simulink model "Radial_KID_MPC"  (R2022a)
settings: Solver=FixedStepAuto  StartTime=0.0  StopTime=Tf  FixedStep=Ts  RelTol=1e-3
values from neighbouring files (symbols this model uses):
  eta = 0.001    [vdp_MPC.m]
  Ts = ts    [dataset_join.m]    (also in vdp_Koopman.m = 0.01)
undefined symbols (not defined in the file or in its folder): DiscIntNeverNeededParam
libraries: sharedTrackingLibrary x1, mpclib x1
settings Model: Creator=sergiovaneg  LastModifiedBy=sergiovaneg

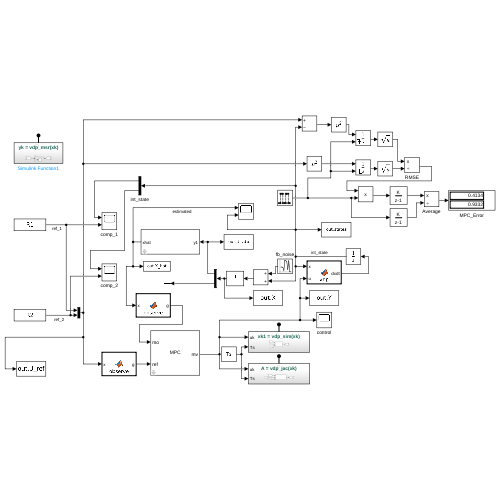
[thumbnail: Simulink's stored preview of the top-level diagram]
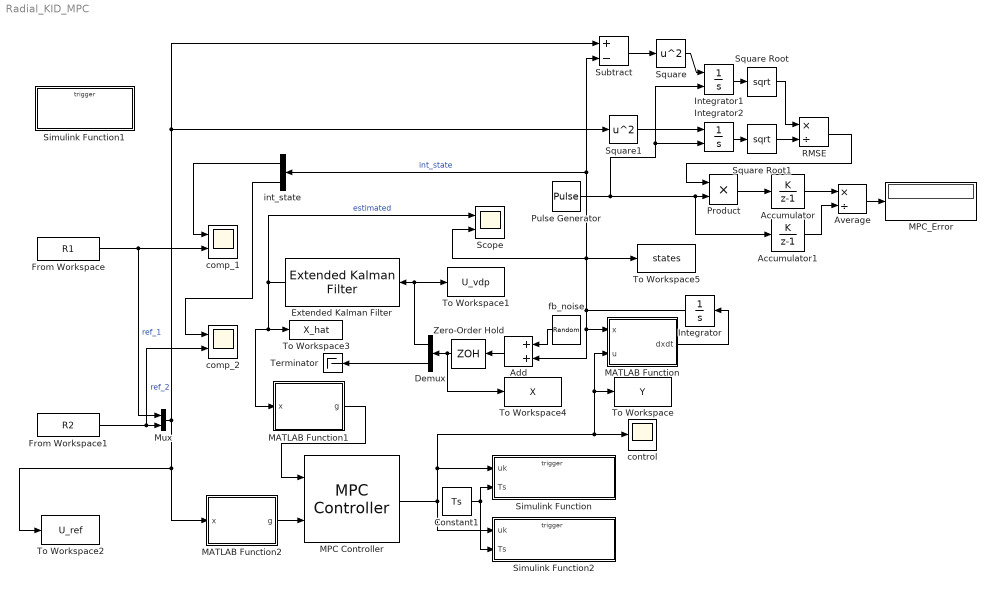
== system Radial_KID_MPC ==
  Accumulator : DiscreteIntegrator  IntegratorMethod=Accumulation: Forward Euler  InitialCondition=[0;0]  SampleTime=Ts  ICPrevOutput=DiscIntNeverNeededParam  ICPrevScaledInput=DiscIntNeverNeededParam
  Accumulator1 : DiscreteIntegrator  IntegratorMethod=Accumulation: Forward Euler  SampleTime=-1  ICPrevOutput=DiscIntNeverNeededParam  ICPrevScaledInput=DiscIntNeverNeededParam
  Add : Sum
  Average : Product  Inputs=*/
  Constant1 : Constant  Value=Ts
  Demux : Demux  Outputs=2
  Extended Kalman Filter : sharedTrackingLibrary/Extended Kalman Filter  StateTransitionFcn=vdp_sim  HasStateTransitionJacobianFcn=on  StateTransitionJacobianFcn=vdp_jac  HasAdditiveProcessNoise=Additive  ProcessNoise=eta  HasTimeVaryingProcessNoise=off  HasStateTransitionFcnExtraArgument=0  InitialState=[0;0]  InitialStateCovariance=eta  MeasurementFcn1=vdp_msr  HasMeasurementJacobianFcn1=off  HasMeasurementEnablePort1=off  HasAdditiveMeasurementNoise1=Additive  MeasurementNoise1=eta  HasTimeVaryingMeasurementNoise1=off  HasMeasurementFcnExtraArgument1=0  HasMeasurementWrapping1=off  MeasurementFcn2=myMeasurementFcn  HasMeasurementJacobianFcn2=off  HasMeasurementEnablePort2=off  HasAdditiveMeasurementNoise2=Additive  MeasurementNoise2=1  HasTimeVaryingMeasurementNoise2=off  HasMeasurementFcnExtraArgument2=0  HasMeasurementWrapping2=off  MeasurementFcn3=myMeasurementFcn  HasMeasurementJacobianFcn3=off  HasMeasurementEnablePort3=off  HasAdditiveMeasurementNoise3=Additive  MeasurementNoise3=1  HasTimeVaryingMeasurementNoise3=off  HasMeasurementFcnExtraArgument3=0  HasMeasurementWrapping3=off  MeasurementFcn4=myMeasurementFcn  HasMeasurementJacobianFcn4=off  HasMeasurementEnablePort4=off  HasAdditiveMeasurementNoise4=Additive  MeasurementNoise4=1  HasTimeVaryingMeasurementNoise4=off  HasMeasurementFcnExtraArgument4=0  HasMeasurementWrapping4=off  MeasurementFcn5=myMeasurementFcn  HasMeasurementJacobianFcn5=off  HasMeasurementEnablePort5=off  HasAdditiveMeasurementNoise5=Additive  MeasurementNoise5=1  HasTimeVaryingMeasurementNoise5=off  HasMeasurementFcnExtraArgument5=0  HasMeasurementWrapping5=off  EnableMultirate=off  StateTransitionFcnSampleTime=1  MeasurementFcn1SampleTime=1  MeasurementFcn2SampleTime=1  MeasurementFcn3SampleTime=1  MeasurementFcn4SampleTime=1  MeasurementFcn5SampleTime=1  UseCurrentEstimator=on  OutputStateCovariance=off  DataType=double  SampleTime=Ts  NumberOfMeasurements=1
      settings: SourceProductBaseCode=TF,AE,PW,CT,DR,ID,LP,NV,AR,RO,RR,UV,VE
  From Workspace : FromWorkspace  VariableName=R1
  From Workspace1 : FromWorkspace  VariableName=R2
  Integrator : Integrator  InitialCondition=[0;0]
  Integrator1 : Integrator  ExternalReset=falling  InitialCondition=[0;0]
  Integrator2 : Integrator  ExternalReset=falling  InitialCondition=[eps;eps]
  MATLAB Function : MATLAB Function  TreatAsAtomicUnit=on
  MATLAB Function1 : MATLAB Function  TreatAsAtomicUnit=on
  MATLAB Function2 : MATLAB Function  TreatAsAtomicUnit=on
  MPC Controller : mpclib/MPC Controller  SCDEnableBlockLinearizationSpecification=on  mpcobj=controller  x0=ctrl_0  is_multiple=0  enable_value=0  return_u0=off  updateMPCinCallerWorkspace=on  md_inport=off  mv_inport=off  uref_inport=off  return_cost=off  return_mvseq=off  return_qpstatus=off  return_xseq=off  return_state=off  return_ovseq=off  state_inport=off  umin_inport=off  umax_inport=off  ymin_inport=off  ymax_inport=off  cc_inport=off  ywt_inport=off  uwt_inport=off  duwt_inport=off  rhoeps_inport=off  pm_inport=off  MaximumP=10  HorizonChoice=FixedHorizon  n_ts=0.01  n_p=25  n_mv=1  n_md=0  n_ud=0  n_mo=7  n_uo=0  BlockDataType=double  SampleTimeInherited=off  switch_inport=off
  MPC_Error : Display
  Mux : Mux  Inputs=2
  Product : Product
  Pulse Generator : DiscretePulseGenerator  Period=10/Ts  SampleTime=Ts
  RMSE : Product  Inputs=*/
  Scope : Scope  NumInputPorts=2
  Simulink Function : Subsystem  TreatAsAtomicUnit=on
  Simulink Function1 : Subsystem  TreatAsAtomicUnit=on
  Simulink Function2 : Subsystem  TreatAsAtomicUnit=on
  Square : Math  Operator=square
  Square Root : Sqrt
  Square Root1 : Sqrt
  Square1 : Math  Operator=square
  Subtract : Sum  Inputs=+-
  Terminator : Terminator
  To Workspace : ToWorkspace  VariableName=Y  SampleTime=Ts
      settings: Save2DSignal=2-D array (concatenate along first dimension)
  To Workspace1 : ToWorkspace  VariableName=U_vdp  SampleTime=Ts
      settings: Save2DSignal=2-D array (concatenate along first dimension)
  To Workspace2 : ToWorkspace  VariableName=U_ref  SampleTime=Ts
      settings: Save2DSignal=2-D array (concatenate along first dimension)
  To Workspace3 : ToWorkspace  VariableName=X_hat  SampleTime=Ts
      settings: Save2DSignal=2-D array (concatenate along first dimension)
  To Workspace4 : ToWorkspace  VariableName=X  SampleTime=Ts
      settings: Save2DSignal=2-D array (concatenate along first dimension)
  To Workspace5 : ToWorkspace  VariableName=states  SampleTime=Ts
      settings: Save2DSignal=2-D array (concatenate along first dimension)
  Zero-Order Hold : ZeroOrderHold  SampleTime=Ts
  comp_1 : Scope  NumInputPorts=2
  comp_2 : Scope  NumInputPorts=2
  control : Scope
  fb_noise : RandomNumber  Variance=eta  Seed=[2;3]  SampleTime=Ts
  int_state : Demux  Outputs=2
  wires:
  int_state/1 -> comp_1/1
  fb_noise/1 -> Add/1
  MPC Controller/1 -> MATLAB Function/2(u), To Workspace/1, control/1, Simulink Function/1(uk), Simulink Function2/1(uk)
  Integrator/1 -> Subtract/2, int_state/1, Scope/2, To Workspace5/1, Add/2, MATLAB Function/1(x)  "int_state"
  From Workspace1/1 -> comp_2/2, Mux/2  "ref_2"
  int_state/2 -> comp_2/1
  MATLAB Function/1(dxdt) -> Integrator/1
  Mux/1 -> To Workspace2/1, MATLAB Function2/1(x), Subtract/1, Square1/1
  Demux/1 -> Extended Kalman Filter/1, To Workspace1/1
  Demux/2 -> Terminator/1
  Extended Kalman Filter/1 -> MATLAB Function1/1(x), To Workspace3/1, Scope/1  "estimated"
  Zero-Order Hold/1 -> To Workspace4/1, Demux/1
  Add/1 -> Zero-Order Hold/1
  Constant1/1 -> Simulink Function/2(Ts), Simulink Function2/2(Ts)
  Subtract/1 -> Square/1
  Square/1 -> Integrator1/1
  From Workspace/1 -> comp_1/2, Mux/1  "ref_1"
  Integrator1/1 -> Square Root/1
  MATLAB Function1/1(g) -> MPC Controller/1
  MATLAB Function2/1(g) -> MPC Controller/2
  Square Root/1 -> RMSE/1
  Integrator2/1 -> Square Root1/1
  Square1/1 -> Integrator2/1
  Square Root1/1 -> RMSE/2
  Pulse Generator/1 -> Accumulator1/1, Product/2, Integrator1/2, Integrator2/2
  Accumulator/1 -> Average/1
  Product/1 -> Accumulator/1
  RMSE/1 -> Product/1
  Accumulator1/1 -> Average/2
  Average/1 -> MPC_Error/1

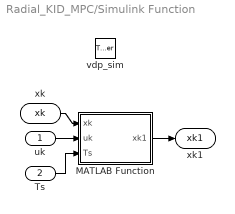
== system Radial_KID_MPC/Simulink Function ==
  uk : Inport
  Ts : Inport  Port=2
  vdp_sim : TriggerPort  TriggerType=function-call  IsSimulinkFunction=on  FunctionName=vdp_sim  FunctionVisibility=scoped  VariantControl=(inherit)
  MATLAB Function : MATLAB Function  TreatAsAtomicUnit=on
  xk : ArgIn  DisableCoverage=on  PortDimensions=2  ArgumentName=xk
  xk1 : ArgOut  DisableCoverage=on  PortDimensions=2  ArgumentName=xk1
  wires:
  xk/1 -> MATLAB Function/1(xk)
  MATLAB Function/1(xk1) -> xk1/1
  uk/1 -> MATLAB Function/2(uk)
  Ts/1 -> MATLAB Function/3(Ts)

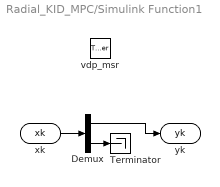
== system Radial_KID_MPC/Simulink Function1 ==
  vdp_msr : TriggerPort  TriggerType=function-call  IsSimulinkFunction=on  FunctionName=vdp_msr  FunctionVisibility=scoped  VariantControl=(inherit)
  Demux : Demux  Outputs=2
  Terminator : Terminator
  xk : ArgIn  DisableCoverage=on  PortDimensions=2  ArgumentName=xk
  yk : ArgOut  DisableCoverage=on  ArgumentName=yk
  wires:
  Demux/2 -> Terminator/1
  xk/1 -> Demux/1
  Demux/1 -> yk/1

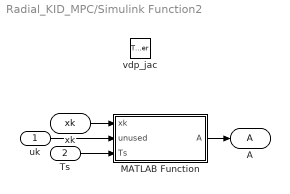
== system Radial_KID_MPC/Simulink Function2 ==
  uk : Inport
  Ts : Inport  Port=2
  vdp_jac : TriggerPort  TriggerType=function-call  IsSimulinkFunction=on  FunctionName=vdp_jac  FunctionVisibility=scoped  VariantControl=(inherit)
  MATLAB Function : MATLAB Function  TreatAsAtomicUnit=on
  xk : ArgIn  DisableCoverage=on  PortDimensions=2  ArgumentName=xk
  A : ArgOut  DisableCoverage=on  PortDimensions=[2 2]  ArgumentName=A
  wires:
  xk/1 -> MATLAB Function/1(xk)
  MATLAB Function/1(A) -> A/1
  uk/1 -> MATLAB Function/2(unused)
  Ts/1 -> MATLAB Function/3(Ts)

== matlab function Radial_KID_MPC/Simulink Function/MATLAB Function ==
  data: xk input; xk1 output; uk input; Ts input
function xk1 = vdp(xk,uk,Ts)
    M = 10;

    delta = Ts/M;
    xk1 = xk;
    for ct=1:M
        xk1 = xk1+delta*vdp_CT0(xk,uk);
    end
end

== matlab function Radial_KID_MPC/MATLAB Function ==
  data: x input; u input; dxdt output
function dxdt = vdp(x,u)
    dxdt = zeros(2,1);
    dxdt(1) = 2*x(2);
    dxdt(2) = -0.8*x(1)+2*x(2)-10*(x(1)^2)*x(2)+u;

== matlab function Radial_KID_MPC/Simulink Function2/MATLAB Function ==
  data: xk input; A output; unused input; Ts input
function A = fcn(xk,~,Ts)
    A=[1,2*Ts;
        Ts*(-0.8-20*xk(1)*xk(2)),1+Ts*(2-xk(1)^2)];
end

== matlab function Radial_KID_MPC/MATLAB Function1 ==
  data: x input; g output; X0 parameter
function g = observe(x,X0)
    g=zeros(size(x,1)+size(X0,2),1);
    aux = vecnorm(X0-x)';
    g(1:size(x,1))=x;
    g(size(x,1)+1:end)=aux.*log(aux.^aux);
end

== matlab function Radial_KID_MPC/MATLAB Function2 ==
  data: x input; g output; X0 parameter
function g = observe(x,X0)
    g=zeros(size(x,1)+size(X0,2),1);
    aux = vecnorm(X0-x)';
    g(1:size(x,1))=x;
    g(size(x,1)+1:end)=aux.*log(aux.^aux);
end
